simulink model "questao1_prova3"  (Simulink 7.9)
settings: Solver=ode45  StartTime=0.0  StopTime=15.0  RelTol=1e-3
settings Model: Creator=Danilo  LastModifiedBy=Danilo

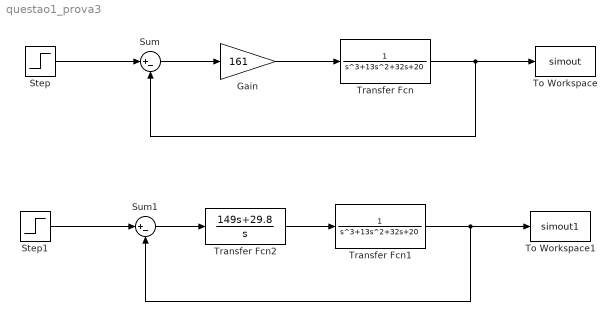
== system questao1_prova3 ==
  Gain : Gain  Gain=161
  Step : Step  Time=0  SampleTime=0
  Step1 : Step  Time=0  SampleTime=0
  Sum : Sum  Inputs=|+-
  Sum1 : Sum  Inputs=|+-
  To Workspace : ToWorkspace  VariableName=simout  SampleTime=-1
  To Workspace1 : ToWorkspace  VariableName=simout1  SampleTime=-1
  Transfer Fcn : TransferFcn  Denominator=[1 13 32 20]
  Transfer Fcn1 : TransferFcn  Denominator=[1 13 32 20]
  Transfer Fcn2 : TransferFcn  Numerator=[149 29.8]  Denominator=[1 0]
  wires:
  Step/1 -> Sum/1
  Sum/1 -> Gain/1
  Gain/1 -> Transfer Fcn/1
  Transfer Fcn/1 -> To Workspace/1, Sum/2
  Step1/1 -> Sum1/1
  Sum1/1 -> Transfer Fcn2/1
  Transfer Fcn2/1 -> Transfer Fcn1/1
  Transfer Fcn1/1 -> To Workspace1/1, Sum1/2
